simulink model "PlantModel"  (R2016a)
settings: Solver=ode45  StartTime=0.0  StopTime=20  RelTol=1e-3
settings Model: Creator=hp  LastModifiedBy=hp

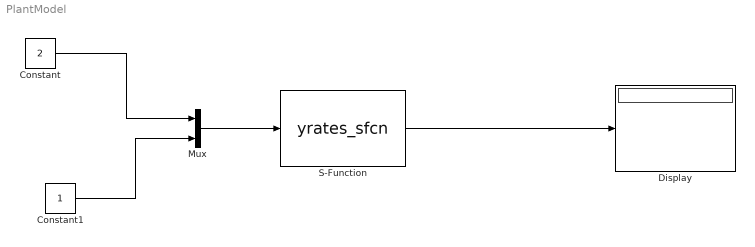
== system PlantModel ==
  Constant : Constant  Value=2
  Constant1 : Constant
  Display : Display
  Mux : Mux  Inputs=2
  S-Function : S-Function  FunctionName=yrates_sfcn  Parameters=Y0  SFunctionDeploymentMode=off  EnableBusSupport=off
  wires:
  Constant/1 -> Mux/1
  Constant1/1 -> Mux/2
  Mux/1 -> S-Function/1
  S-Function/1 -> Display/1
